simulink library "cpid"  (Simulink 8.1)
settings: Solver=ode1  StartTime=0.0  StopTime=Inf  FixedStep=0.001  RelTol=1e-3
PostLoadFcn:
  | , if any(exist('dsrtsu_mdlpostloadfcn', 'file') == [2, 3, 6]), try dsrtsu_mdlpostloadfcn('Execute', bdroot); catch fprintf('Error in PostLoadFcn (dsrtsu_mdlpostloadfcn) for model "%s":\n %s\n', bdroot, lasterr); end, end,
libraries: cft x1, cst x1
settings Model: DSRTSU_INTERNAL_RTI_VER=450  DSRTSU_INTERNAL_RTI_TYPE=rti1401  RTICANMMDATA=struct('GeneralSetupData',struct('modelroot','D:\Projects\ELN150201\Repositories\Taiwan\trunk\AdasDragon\software\sw_development\arch\app\jud','generalsettings',struct('filesettings',struct('destfolder',struct('Name','RTICANMM_FILES','Check',1),'buildfolder',struct('Name','.','Check',1),'AbsDestfolder',struct('Name','D:\Projects\ELN150201\Repositories\Taiwan\trunk\AdasDragon\software\sw_development\arch\app\jud\RTICANMM_FILES'),'AbsBuildfolder',struct('Name','D:\Projects\ELN150201\Repositories\Taiwan\trunk\AdasDragon\software\sw_development\arch\app\jud'))),'options',struct('addpaths',1,'rmpaths',1,'addtrcexclusion',logical(1),'cannavigator',struct('checkmonitoring',0),'show_usrtrc',0,'use_usrtrc',0),'advanced',struct('options',[1 1 1 1 1 1 1 1 1 1 1 1 1 1 1 1 1 1 1 1 1 1 1 1 1 1 1 1 1 1 1 1 1 1 1 1 1 1 1 1 1 1 1 1 1 1 1 1 1 1 1 1 1 1 1 1 1 1 1 1 1 1 1 1 1 1 1 1 1 1 1 1 1 1 1 1 1 1 1 1 1 1 1 1 1 1 1 1 1 1 1 1 1 1 1 1 1 1 1 1]),'MPSetup',{{}},'modelname','cpid','block','cpid'))  DSRTSU_INTERNAL_RTIFPGA=40  Creator=AT015411  LastModifiedBy=AT015086

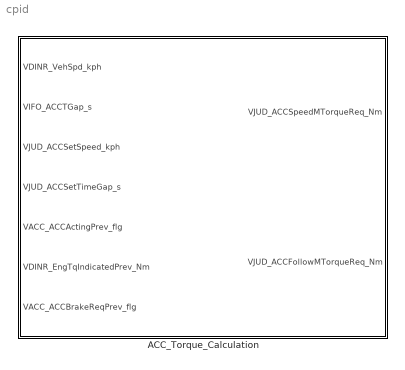
== system cpid ==
  ACC_Torque_Calculation : Subsystem

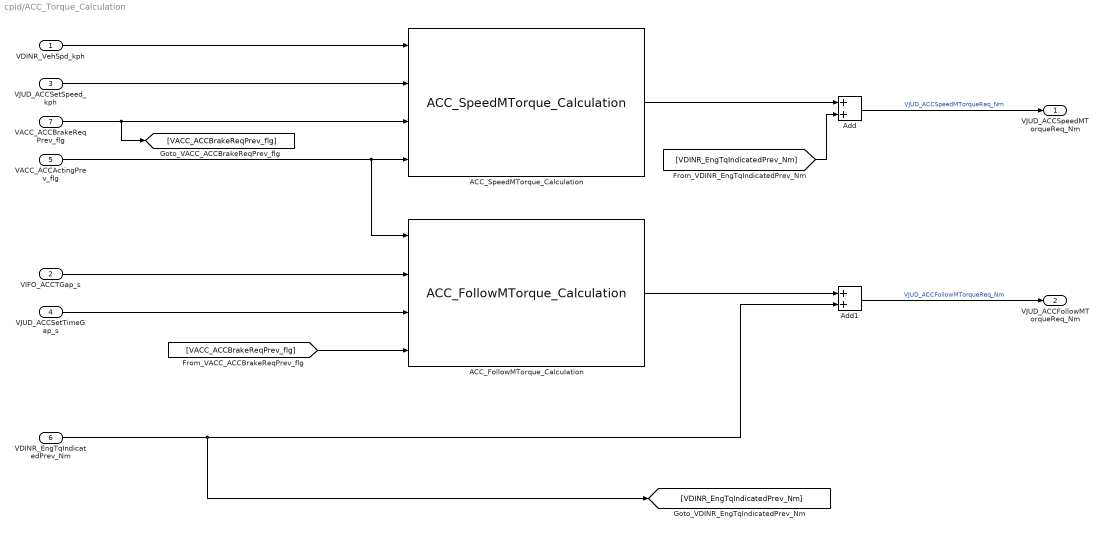
== system cpid/ACC_Torque_Calculation ==
  VDINR_VehSpd_kph : Inport
  VIFO_ACCTGap_s : Inport  Port=2
  VJUD_ACCSetSpeed_kph : Inport  Port=3
  VJUD_ACCSetTimeGap_s : Inport  Port=4
  VACC_ACCActingPrev_flg : Inport  Port=5
  VDINR_EngTqIndicatedPrev_Nm : Inport  Port=6
  VACC_ACCBrakeReqPrev_flg : Inport  Port=7
  ACC_FollowMTorque_Calculation : cft/ACC_FollowMTorque_Calculation
  ACC_SpeedMTorque_Calculation : cst/ACC_SpeedMTorque_Calculation
  Add : Sum
  Add1 : Sum
  VJUD_ACCSpeedMTorqueReq_Nm : Outport
  VJUD_ACCFollowMTorqueReq_Nm : Outport  Port=2
  wires:
  [VACC_ACCBrakeReqPrev_flg] -> ACC_FollowMTorque_Calculation/4
  VACC_ACCBrakeReqPrev_flg/1 -> [VACC_ACCBrakeReqPrev_flg], ACC_SpeedMTorque_Calculation/3
  ACC_FollowMTorque_Calculation/1 -> Add1/1
  ACC_SpeedMTorque_Calculation/1 -> Add/1
  [VDINR_EngTqIndicatedPrev_Nm] -> Add/2
  VDINR_EngTqIndicatedPrev_Nm/1 -> [VDINR_EngTqIndicatedPrev_Nm], Add1/2
  VACC_ACCActingPrev_flg/1 -> ACC_FollowMTorque_Calculation/1, ACC_SpeedMTorque_Calculation/4
  VIFO_ACCTGap_s/1 -> ACC_FollowMTorque_Calculation/2
  VJUD_ACCSetTimeGap_s/1 -> ACC_FollowMTorque_Calculation/3
  Add1/1 -> VJUD_ACCFollowMTorqueReq_Nm/1  "VJUD_ACCFollowMTorqueReq_Nm"
  VJUD_ACCSetSpeed_kph/1 -> ACC_SpeedMTorque_Calculation/2
  Add/1 -> VJUD_ACCSpeedMTorqueReq_Nm/1  "VJUD_ACCSpeedMTorqueReq_Nm"
  VDINR_VehSpd_kph/1 -> ACC_SpeedMTorque_Calculation/1
